simulink model "Book4341"  (R2019b)
settings: Solver=ode4  StartTime=0.001  StopTime=30  FixedStep=0.001  RelTol=1e-3
settings Model: Creator=xyh  LastModifiedBy=user

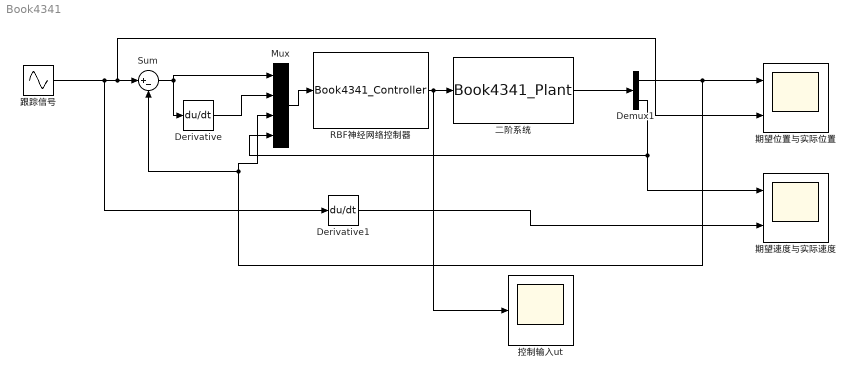
== system Book4341 ==
  Demux1 : Demux  Outputs=2
  Derivative : Derivative
  Derivative1 : Derivative
  Mux : Mux
  RBF神经网络控制器 : S-Function  FunctionName=Book4341_Controller  SFunctionDeploymentMode=off  EnableBusSupport=off
  Sum : Sum  Inputs=|+-
  二阶系统 : S-Function  FunctionName=Book4341_Plant  SFunctionDeploymentMode=off  EnableBusSupport=off
  控制输入ut : Scope
  期望位置与实际位置 : Scope  NumInputPorts=2
  期望速度与实际速度 : Scope  NumInputPorts=2
  跟踪信号 : Sin  SampleTime=0
  wires:
  RBF神经网络控制器/1 -> 控制输入ut/1, 二阶系统/1
  Derivative/1 -> Mux/2
  Sum/1 -> Derivative/1, Mux/1
  Derivative1/1 -> 期望速度与实际速度/2
  Demux1/1 -> 期望位置与实际位置/1, Sum/2, Mux/3
  二阶系统/1 -> Demux1/1
  Mux/1 -> RBF神经网络控制器/1
  Demux1/2 -> 期望速度与实际速度/1, Mux/4
  跟踪信号/1 -> Derivative1/1, Sum/1, 期望位置与实际位置/2
